simulink library "DesiredStateSelector"  (R2016b)
settings: Solver=VariableStepAuto  StartTime=0.0  StopTime=10.0  RelTol=1e-3
settings Model: Creator=march  LastModifiedBy=MARCH

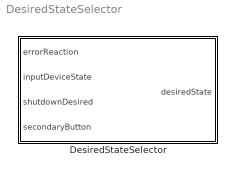
== system DesiredStateSelector ==
  DesiredStateSelector : Subsystem

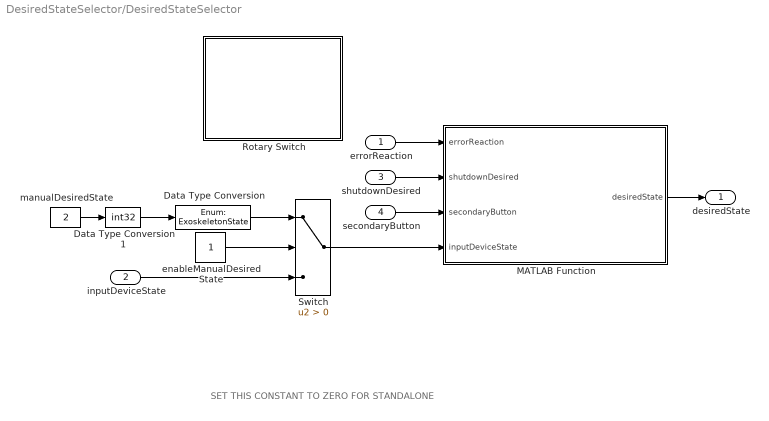
== system DesiredStateSelector/DesiredStateSelector ==
  note: SET THIS CONSTANT TO ZERO FOR STANDALONE
  errorReaction : Inport
  inputDeviceState : Inport  Port=2
  shutdownDesired : Inport  Port=3
  secondaryButton : Inport  Port=4
  Data Type Conversion : DataTypeConversion  OutDataTypeStr=Enum: ExoskeletonState
  Data Type Conversion1 : DataTypeConversion  OutDataTypeStr=int32
  MATLAB Function : MATLAB Function  TreatAsAtomicUnit=on
  Rotary Switch : Subsystem  DialogController=hmiCreateDDGDialog  IsWebBlock=on  mask(MWDashboardBlock){webBlockId=4bc12d98-0fca-4dce-957e-1bb7b079bead, webBlockType=discreteknob, ShowInLibBrowser=on, ShowInitialText=on, HMISrcModelName=DesiredStateSelector}
      mask prompts: webBlockId "WebBlock Id"; webBlockType "WebBlock Type"; HMISrcModelName "Source Model"
      mask help: SimulinkHMI:dialogs:DiscreteKnobDialogDesc
      mask Help: helpview([docroot '/mapfiles/simulink.map'], 'hmi_rotary_switch')
      mask Display:
      | model = bdroot(gcb);
      | if strcmp(get_param(model,'BlockDiagramType'), 'library')
      |     image([(matlabroot) '/toolbox/simulink/hmi/icons/DiscreteKnob.png']);
      | end
  Switch : Switch  Criteria=u2 > Threshold
  enableManualDesiredState : Constant
  manualDesiredState : Constant  Value=2
  desiredState : Outport
  wires:
  errorReaction/1 -> MATLAB Function/1(errorReaction)
  secondaryButton/1 -> MATLAB Function/3(secondaryButton)
  manualDesiredState/1 -> Data Type Conversion1/1
  Data Type Conversion/1 -> Switch/1
  Data Type Conversion1/1 -> Data Type Conversion/1
  enableManualDesiredState/1 -> Switch/2
  Switch/1 -> MATLAB Function/4(inputDeviceState)
  inputDeviceState/1 -> Switch/3
  MATLAB Function/1(desiredState) -> desiredState/1
  shutdownDesired/1 -> MATLAB Function/2(shutdownDesired)

== system DesiredStateSelector/DesiredStateSelector/Rotary Switch ==

== matlab function DesiredStateSelector/MATLAB Function ==
  data: errorReaction input; shutdownDesired input; desiredState output; secondaryButton input; inputDeviceState input
function desiredState = getDesiredState( errorReaction, shutdownDesired, secondaryButton, inputDeviceState )
% wrapper function for getDesiredState
desiredState = getDesiredState( errorReaction, shutdownDesired, secondaryButton, inputDeviceState );
end
